simulink model "TST_Diff_PlausPrtTrq"  (R2016b)
settings: Solver=FixedStepDiscrete  StartTime=0.0  StopTime=simTime  FixedStep=sampleTime  RelTol=1e-3
values from neighbouring files (symbols this model uses):
  testCase = 1    [initTST_Diff_PlausPrtTrq_001.m]
libraries: simulink x3, UnitTest_Lib x1
settings Model: Creator=zhengjinyan  LastModifiedBy=zhengjinyan
settings DebuggingCC: SignalRangeChecking=error

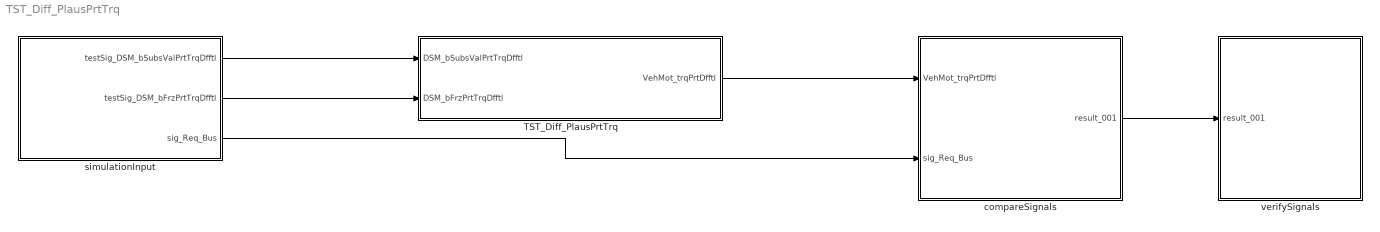
== system TST_Diff_PlausPrtTrq ==
  TST_Diff_PlausPrtTrq : Subsystem
  compareSignals : Subsystem
  simulationInput : Subsystem
  verifySignals : Subsystem
  wires:
  simulationInput/1(testSig_DSM_bSubsValPrtTrqDfftl) -> TST_Diff_PlausPrtTrq/1(DSM_bSubsValPrtTrqDfftl)
  simulationInput/2(testSig_DSM_bFrzPrtTrqDfftl) -> TST_Diff_PlausPrtTrq/2(DSM_bFrzPrtTrqDfftl)
  TST_Diff_PlausPrtTrq/1(VehMot_trqPrtDfftl) -> compareSignals/1(VehMot_trqPrtDfftl)
  simulationInput/3(sig_Req_Bus) -> compareSignals/2(sig_Req_Bus)
  compareSignals/1(result_001) -> verifySignals/1(result_001)

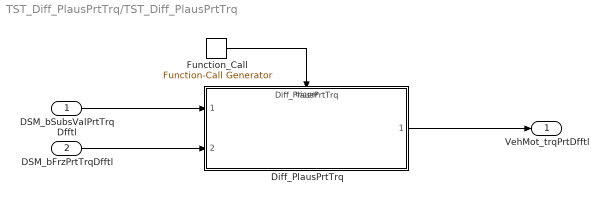
== system TST_Diff_PlausPrtTrq/TST_Diff_PlausPrtTrq ==
  DSM_bSubsValPrtTrqDfftl : Inport
  DSM_bFrzPrtTrqDfftl : Inport  Port=2
  Diff_PlausPrtTrq : ModelReference  ModelNameDialog=Diff_PlausPrtTrq  SimulationMode=Normal  ModelReferenceVersion=1.11  TriggerPortName=function  TriggerPortTriggerType=function-call  TriggerPortStatesWhenEnabling=held
  Function_Call : simulink/Ports & Subsystems/Function-Call Generator  sample_time=sampleTime  numberOfIterations=1
  VehMot_trqPrtDfftl : Outport
  wires:
  Function_Call/1 -> Diff_PlausPrtTrq/Trigger
  DSM_bSubsValPrtTrqDfftl/1 -> Diff_PlausPrtTrq/1
  DSM_bFrzPrtTrqDfftl/1 -> Diff_PlausPrtTrq/2
  Diff_PlausPrtTrq/1 -> VehMot_trqPrtDfftl/1

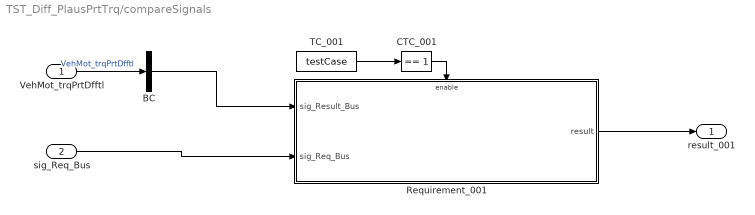
== system TST_Diff_PlausPrtTrq/compareSignals ==
  VehMot_trqPrtDfftl : Inport
  sig_Req_Bus : Inport  Port=2
  BC : BusCreator  Inputs=1
  CTC_001 : simulink/Logic and Bit Operations/Compare To Constant  relop===  const=1  OutDataTypeStr=boolean
  Requirement_001 : Subsystem
  TC_001 : Constant  Value=testCase
  result_001 : Outport
  wires:
  VehMot_trqPrtDfftl/1 -> BC/1  "VehMot_trqPrtDfftl"
  TC_001/1 -> CTC_001/1
  CTC_001/1 -> Requirement_001/Enable
  sig_Req_Bus/1 -> Requirement_001/2(sig_Req_Bus)
  BC/1 -> Requirement_001/1(sig_Result_Bus)
  Requirement_001/1(result) -> result_001/1

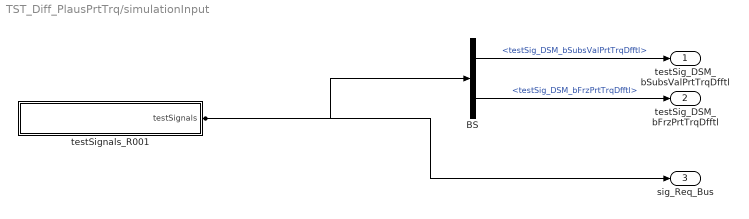
== system TST_Diff_PlausPrtTrq/simulationInput ==
  BS : BusSelector  OutputSignals=testSig_DSM_bSubsValPrtTrqDfftl,testSig_DSM_bFrzPrtTrqDfftl
  testSignals_R001 : Subsystem
  testSig_DSM_bSubsValPrtTrqDfftl : Outport
  testSig_DSM_bFrzPrtTrqDfftl : Outport  Port=2
  sig_Req_Bus : Outport  Port=3
  wires:
  BS/1 -> testSig_DSM_bSubsValPrtTrqDfftl/1  "<testSig_DSM_bSubsValPrtTrqDfftl>"
  BS/2 -> testSig_DSM_bFrzPrtTrqDfftl/1  "<testSig_DSM_bFrzPrtTrqDfftl>"
  testSignals_R001/1(testSignals) -> BS/1, sig_Req_Bus/1

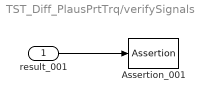
== system TST_Diff_PlausPrtTrq/verifySignals ==
  result_001 : Inport
  Assertion_001 : Assertion  Enabled=off
  wires:
  result_001/1 -> Assertion_001/1

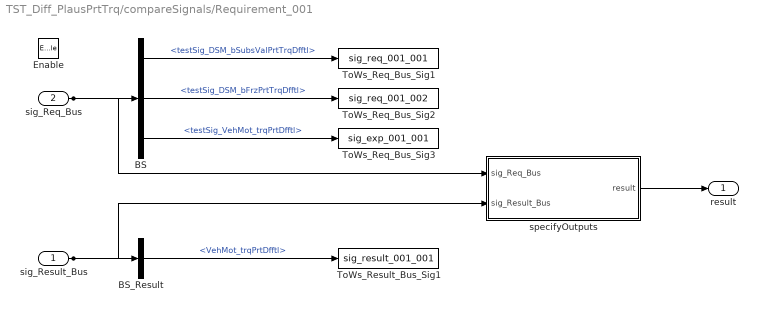
== system TST_Diff_PlausPrtTrq/compareSignals/Requirement_001 ==
  sig_Result_Bus : Inport
  sig_Req_Bus : Inport  Port=2
  Enable : EnablePort
  BS : BusSelector  OutputSignals=testSig_DSM_bSubsValPrtTrqDfftl,testSig_DSM_bFrzPrtTrqDfftl,testSig_VehMot_trqPrtDfftl
  BS_Result : BusSelector  OutputSignals=VehMot_trqPrtDfftl
  ToWs_Req_Bus_Sig1 : ToWorkspace  VariableName=sig_req_001_001  SaveFormat=Structure With Time
  ToWs_Req_Bus_Sig2 : ToWorkspace  VariableName=sig_req_001_002  SaveFormat=Structure With Time
  ToWs_Req_Bus_Sig3 : ToWorkspace  VariableName=sig_exp_001_001  SaveFormat=Structure With Time
  ToWs_Result_Bus_Sig1 : ToWorkspace  VariableName=sig_result_001_001  SaveFormat=Structure With Time
  specifyOutputs : Subsystem
  result : Outport
  wires:
  sig_Req_Bus/1 -> BS/1, specifyOutputs/1(sig_Req_Bus)
  BS/1 -> ToWs_Req_Bus_Sig1/1  "<testSig_DSM_bSubsValPrtTrqDfftl>"
  BS/2 -> ToWs_Req_Bus_Sig2/1  "<testSig_DSM_bFrzPrtTrqDfftl>"
  BS/3 -> ToWs_Req_Bus_Sig3/1  "<testSig_VehMot_trqPrtDfftl>"
  sig_Result_Bus/1 -> BS_Result/1, specifyOutputs/2(sig_Result_Bus)
  BS_Result/1 -> ToWs_Result_Bus_Sig1/1  "<VehMot_trqPrtDfftl>"
  specifyOutputs/1(result) -> result/1

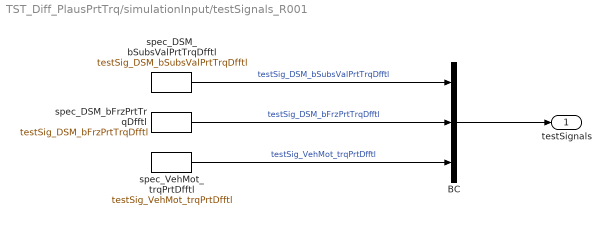
== system TST_Diff_PlausPrtTrq/simulationInput/testSignals_R001 ==
  BC : BusCreator  Inputs=3
  spec_DSM_bFrzPrtTrqDfftl : FromWorkspace  VariableName=testSig_DSM_bFrzPrtTrqDfftl  Interpolate=off  OutputAfterFinalValue=Holding final value
  spec_DSM_bSubsValPrtTrqDfftl : FromWorkspace  VariableName=testSig_DSM_bSubsValPrtTrqDfftl  Interpolate=off  OutputAfterFinalValue=Holding final value
  spec_VehMot_trqPrtDfftl : FromWorkspace  VariableName=testSig_VehMot_trqPrtDfftl  Interpolate=off  OutputAfterFinalValue=Holding final value
  testSignals : Outport
  wires:
  BC/1 -> testSignals/1
  spec_DSM_bSubsValPrtTrqDfftl/1 -> BC/1  "testSig_DSM_bSubsValPrtTrqDfftl"
  spec_DSM_bFrzPrtTrqDfftl/1 -> BC/2  "testSig_DSM_bFrzPrtTrqDfftl"
  spec_VehMot_trqPrtDfftl/1 -> BC/3  "testSig_VehMot_trqPrtDfftl"

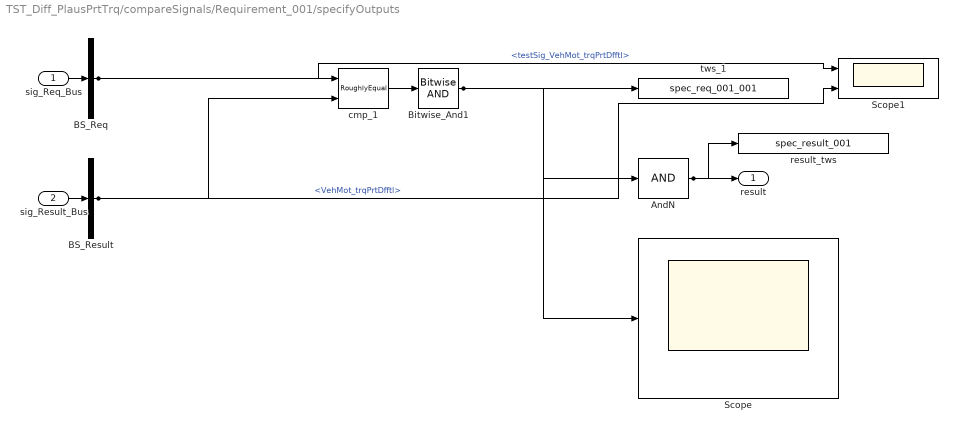
== system TST_Diff_PlausPrtTrq/compareSignals/Requirement_001/specifyOutputs ==
  sig_Req_Bus : Inport
  sig_Result_Bus : Inport  Port=2
  AndN : Logic  Inputs=1
  BS_Req : BusSelector  OutputSignals=testSig_VehMot_trqPrtDfftl
  BS_Result : BusSelector  OutputSignals=VehMot_trqPrtDfftl
  Bitwise_And1 : simulink/Logic and Bit Operations/Bitwise Operator  logicop=AND  UseBitMask=off  BitMask=bin2dec('11011001')  BitMaskRealWorld=Stored Integer
  Scope : Scope
  Scope1 : Scope  NumInputPorts=2
  cmp_1 : UnitTest_Lib/RoughlyEqual  slope=0.1
  result_tws : ToWorkspace  VariableName=spec_result_001
  tws_1 : ToWorkspace  VariableName=spec_req_001_001
  result : Outport
  wires:
  sig_Req_Bus/1 -> BS_Req/1
  sig_Result_Bus/1 -> BS_Result/1
  AndN/1 -> result/1, result_tws/1
  BS_Req/1 -> cmp_1/1, Scope1/1  "<testSig_VehMot_trqPrtDfftl>"
  BS_Result/1 -> cmp_1/2, Scope1/2  "<VehMot_trqPrtDfftl>"
  cmp_1/1 -> Bitwise_And1/1
  Bitwise_And1/1 -> tws_1/1, AndN/1, Scope/1
